simulink model "s5b"  (Simulink 2.00)
settings: Solver=ode15s  StartTime=0.0  StopTime=tstop  MaxStep=5e-3  RelTol=5e-6  AbsTol=1e-6
values from neighbouring files (symbols this model uses):
  Domega = 0    [P1HP.M]    (also in PSPH.M)
  H = J*wbm*wbm/(2*Sb)    (= 2.36870505626)    [P1HP.M]    (also in PSPH.M = 1.39074103839)
  Psidso = 0    [M1.M]    (also in M4.M; M4STP.M; M5.M)
  Psipdro = 0    [M1.M]    (also in M4.M; M4STP.M; M5.M; M6.M)
  Psipqro = 0    [M1.M]    (also in M4.M = Vm; M4STP.M = Vm; M5.M; M6.M)
  Psiqso = 0    [M1.M]    (also in M4.M = Vm; M4STP.M = Vm; M5.M; M6.M)
  rpr = 1.99    [P1HP.M]    (also in PSPH.M = 4.12)
  rs = 3.35    [P1HP.M]
  Tb = Sb/wbm    (= 3.9788735773)    [P1HP.M]    (also in PSPH.M = 0.989413229555)
  Tfactor = (3*P)/(4*wb)    (= 0.00795774715459)    [P1HP.M]    (also in PSPH.M = 0.00530516476973)
  Vm = Vrated*sqrt(2/3)    [M4.M]    (also in P1HP.M; PSPH.M = Vrated*sqrt(2))
  wb = 2*pi*frated    (= 376.991118431)    [P1HP.M]    (also in PSPH.M)
  wrbywbo = 0    [M1.M]    (also in M4.M = 1; M4STP.M = 1; M5.M; M6.M)
  xls = 6.94e-3*wb    (= 2.61631836191)    [P1HP.M]
  xM = 1/(1/xm + 1/xls + 1/xplr)    (= 1.2810101836)    [P1HP.M]
  xplr = xls    (= 2.61631836191)    [P1HP.M]    (also in PSPH.M = 2.12)
  Zb = Vrated*Vrated/Sb    (= 53.3333333333)    [P1HP.M]    (also in PSPH.M = 64.8793565684)
settings Model: MaxOrder=3  SaveTime=off  SaveOutput=off  ConsistencyChecking=off

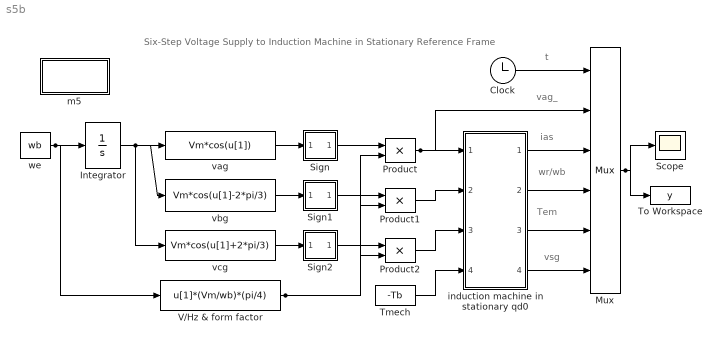
== system s5b ==
  note: Six-Step Voltage Supply to Induction Machine
      | in Stationary Reference Frame
  note: wr/wb
  note: Tem
  note: vsg
  note: ias
  note: vag_
  note: t
  Clock : Clock
      settings: DeleteFcn=simclock BlockIsBeingDestroyed  PostSaveFcn=simclock Save
  Integrator : Integrator  ExternalReset=none  InitialConditionSource=internal  InitialCondition=0  LimitOutput=off  UpperSaturationLimit=inf  LowerSaturationLimit=-inf  ShowSaturationPort=off  ShowStatePort=off  AbsoluteTolerance=auto
  m5 : Subsystem
      settings: OpenFcn=m5
      mask Type: Masked block of m5.m
      mask Help: Uses m5.5 to initialize and plot
      mask Display: disp('Initialize\nand plot')
  Mux : Mux  Inputs=6
  Product : Product  Inputs=2
  Product1 : Product  Inputs=2
  Product2 : Product  Inputs=2
  Scope : Scope
      settings: TickLabels=on  TimeRange=2  YMin=-20  YMax=20  SaveToWorkspace=off  SaveName=ScopeData  LimitMaxRows=off  Decimation=2
  Sign : Subsystem
      mask Type: Sign
      mask Description: y = sign(x)
      mask Help: Sign Function:\n\t\t\ty = 1 if x > 0\n\t\t\ty = 0 if x = 0\n\t\t\ty = -1 if x < 0
      mask Display: plot(-50,-50,50,50,[-50,50],[0,0],[0,0],[-50,50],[-40,0],[-30,-30],[0,40],[30,30])
  Sign1 : Subsystem
      mask Type: Sign
      mask Description: y = sign(x)
      mask Help: Sign Function:\n\t\t\ty = 1 if x > 0\n\t\t\ty = 0 if x = 0\n\t\t\ty = -1 if x < 0
      mask Display: plot(-50,-50,50,50,[-50,50],[0,0],[0,0],[-50,50],[-40,0],[-30,-30],[0,40],[30,30])
  Sign2 : Subsystem
      mask Type: Sign
      mask Description: y = sign(x)
      mask Help: Sign Function:\n\t\t\ty = 1 if x > 0\n\t\t\ty = 0 if x = 0\n\t\t\ty = -1 if x < 0
      mask Display: plot(-50,-50,50,50,[-50,50],[0,0],[0,0],[-50,50],[-40,0],[-30,-30],[0,40],[30,30])
  Tmech : Constant  Value=-Tb
  To Workspace : ToWorkspace  VariableName=y  SampleTime=0
      settings: Buffer=50000
  V/Hz & form factor : Fcn  Expr=u[1]*(Vm/wb)*(pi/4)
  induction machine in stationary qd0 : Subsystem
  vag : Fcn  Expr=Vm*cos(u[1])
  vbg : Fcn  Expr=Vm*cos(u[1]-2*pi/3)
  vcg : Fcn  Expr=Vm*cos(u[1]+2*pi/3)
  we : Constant  Value=wb
  wires:
  V/Hz & form factor/1 -> Product1/2, Product/2, Product2/2
  we/1 -> V/Hz & form factor/1, Integrator/1
  vcg/1 -> Sign2/1(in_1)
  vbg/1 -> Sign1/1(in_1)
  vag/1 -> Sign/1(in_1)
  Integrator/1 -> vbg/1, vag/1, vcg/1
  induction machine in stationary qd0/4(out_vsg) -> Mux/6
  induction machine in stationary qd0/3(out_Tem) -> Mux/5
  induction machine in stationary qd0/2(out_wr/wb) -> Mux/4
  induction machine in stationary qd0/1(out_ias) -> Mux/3
  Tmech/1 -> induction machine in stationary qd0/4(in_Tmech)
  Product/1 -> Mux/2, induction machine in stationary qd0/1(in_vag)
  Sign2/1(out_1) -> Product2/1
  Sign1/1(out_1) -> Product1/1
  Sign/1(out_1) -> Product/1
  Product2/1 -> induction machine in stationary qd0/3(in_vcg)
  Product1/1 -> induction machine in stationary qd0/2(in_vbg)
  Clock/1 -> Mux/1
  Mux/1 -> Scope/1, To Workspace/1

== system s5b/m5 ==
  note: Uses m5.m to initIalize simulation
      | and plot results

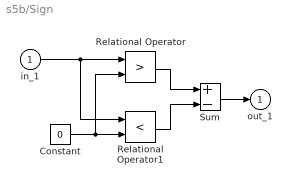
== system s5b/Sign ==
  in_1 : Inport  Port=1  PortWidth=-1  SampleTime=-1
  Constant : Constant  Value=0
  Relational Operator : RelationalOperator  Operator=>
  Relational Operator1 : RelationalOperator  Operator=<
  Sum : Sum  Inputs=+-
  out_1 : Outport  Port=1  InitialOutput=0
  wires:
  Sum/1 -> out_1/1
  Relational Operator/1 -> Sum/1
  Relational Operator1/1 -> Sum/2
  Constant/1 -> Relational Operator/2, Relational Operator1/2
  in_1/1 -> Relational Operator1/1, Relational Operator/1

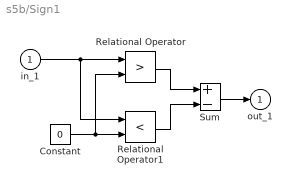
== system s5b/Sign1 ==
  in_1 : Inport  Port=1  PortWidth=-1  SampleTime=-1
  Constant : Constant  Value=0
  Relational Operator : RelationalOperator  Operator=>
  Relational Operator1 : RelationalOperator  Operator=<
  Sum : Sum  Inputs=+-
  out_1 : Outport  Port=1  InitialOutput=0
  wires:
  Sum/1 -> out_1/1
  Relational Operator/1 -> Sum/1
  Relational Operator1/1 -> Sum/2
  Constant/1 -> Relational Operator/2, Relational Operator1/2
  in_1/1 -> Relational Operator1/1, Relational Operator/1

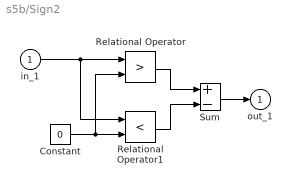
== system s5b/Sign2 ==
  in_1 : Inport  Port=1  PortWidth=-1  SampleTime=-1
  Constant : Constant  Value=0
  Relational Operator : RelationalOperator  Operator=>
  Relational Operator1 : RelationalOperator  Operator=<
  Sum : Sum  Inputs=+-
  out_1 : Outport  Port=1  InitialOutput=0
  wires:
  Sum/1 -> out_1/1
  Relational Operator/1 -> Sum/1
  Relational Operator1/1 -> Sum/2
  Constant/1 -> Relational Operator/2, Relational Operator1/2
  in_1/1 -> Relational Operator1/1, Relational Operator/1

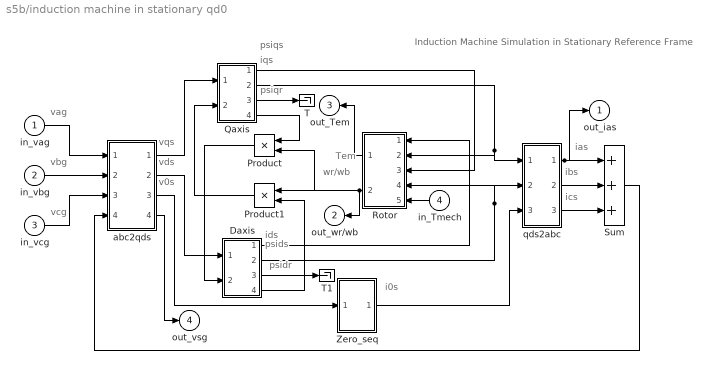
== system s5b/induction machine in stationary qd0 ==
  note: vbg
  note: ids
  note: v0s
  note: vds
  note: vqs
  note: ias
  note: psidr
  note: psids
  note: ics
  note: ibs
  note: psiqr
  note: iqs
  note: psiqs
  note: wr/wb
  note: Tem
  note: vcg
  note: vag
  note: i0s
  note: Induction Machine Simulation
      |   in Stationary Reference Frame
  in_vag : Inport  Port=1  PortWidth=-1  SampleTime=-1
  in_vbg : Inport  Port=2  PortWidth=-1  SampleTime=-1
  in_vcg : Inport  Port=3  PortWidth=-1  SampleTime=-1
  in_Tmech : Inport  Orientation=left  Port=4  PortWidth=-1  SampleTime=-1
  Daxis : Subsystem
  Product : Product  Orientation=left  Inputs=2
  Product1 : Product  Orientation=left  Inputs=2
  Qaxis : Subsystem
  Rotor : Subsystem  Orientation=left
  Sum : Sum  Inputs=+++
  T : Terminator
  T1 : Terminator
  Zero_seq : Subsystem
  abc2qds : Subsystem
  qds2abc : Subsystem
  out_ias : Outport  Port=1  InitialOutput=0
  out_wr/wb : Outport  Orientation=left  Port=2  InitialOutput=0
  out_Tem : Outport  Orientation=left  Port=3  InitialOutput=0
  out_vsg : Outport  Port=4  InitialOutput=0
  wires:
  Daxis/3(out_idr') -> T1/1
  Qaxis/3(out_iqr') -> T/1
  abc2qds/4(out_vsg) -> out_vsg/1
  in_Tmech/1 -> Rotor/5(in_Tmech)
  in_vcg/1 -> abc2qds/3(in_vcg)
  in_vbg/1 -> abc2qds/2(in_vbg)
  qds2abc/1(out_ias) -> out_ias/1, Sum/1
  Rotor/1(out_Tem) -> out_Tem/1
  in_vag/1 -> abc2qds/1(in_vag)
  Daxis/2(out_ids) -> Rotor/4(in_ids), qds2abc/2(in_ids)
  Product1/1 -> Qaxis/2(in_(wr/wb)*psidr')
  Qaxis/1(out_psiqs) -> Rotor/3(in_psiqs)
  abc2qds/2(out_vds) -> Daxis/1(in_vds)
  abc2qds/1(out_vqs) -> Qaxis/1(in_vqs)
  Qaxis/2(out_iqs) -> Rotor/2(in_iqs), qds2abc/1(in_iqs)
  Product/1 -> Daxis/2(in_(wr/wb)*psiqr')
  Daxis/1(out_psids) -> Rotor/1(in_psids)
  Rotor/2(out_wr/wb) -> out_wr/wb/1, Product/2, Product1/1
  Qaxis/4(out_psiqr') -> Product/1
  Daxis/4(out_psidr') -> Product1/2
  abc2qds/3(out_v0s) -> Zero_seq/1(in_v0s)
  qds2abc/2(out_ibs) -> Sum/2
  qds2abc/3(out_ics) -> Sum/3
  Zero_seq/1(out_i0s) -> qds2abc/3(in_i0s)
  Sum/1 -> abc2qds/4(ias+ibs+ics)

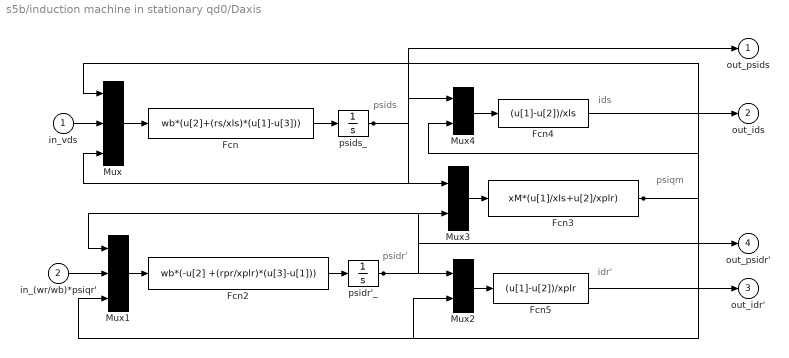
== system s5b/induction machine in stationary qd0/Daxis ==
  note: psidr'
  note: idr'
  note: psiqm
  note: psids
  note: ids
  in_vds : Inport  Port=1  PortWidth=-1  SampleTime=-1
  in_(wr/wb)*psiqr' : Inport  Port=2  PortWidth=-1  SampleTime=-1
  Fcn : Fcn  Expr=wb*(u[2]+(rs/xls)*(u[1]-u[3]))
  Fcn2 : Fcn  Expr=wb*(-u[2] +(rpr/xplr)*(u[3]-u[1]))
  Fcn3 : Fcn  Expr=xM*(u[1]/xls+u[2]/xplr)
  Fcn4 : Fcn  Expr=(u[1]-u[2])/xls
  Fcn5 : Fcn  Expr=(u[1]-u[2])/xplr
  Mux : Mux  Inputs=3
  Mux1 : Mux  Inputs=3
  Mux2 : Mux  Inputs=2
  Mux3 : Mux  Inputs=2
  Mux4 : Mux  Inputs=2
  psidr'_ : Integrator  ExternalReset=none  InitialConditionSource=internal  InitialCondition=Psipdro  LimitOutput=off  UpperSaturationLimit=inf  LowerSaturationLimit=-inf  ShowSaturationPort=off  ShowStatePort=off  AbsoluteTolerance=auto
  psids_ : Integrator  ExternalReset=none  InitialConditionSource=internal  InitialCondition=Psidso  LimitOutput=off  UpperSaturationLimit=inf  LowerSaturationLimit=-inf  ShowSaturationPort=off  ShowStatePort=off  AbsoluteTolerance=auto
  out_psids : Outport  Port=1  InitialOutput=0
  out_ids : Outport  Port=2  InitialOutput=0
  out_idr' : Outport  Port=3  InitialOutput=0
  out_psidr' : Outport  Port=4  InitialOutput=0
  wires:
  Fcn5/1 -> out_idr'/1
  in_(wr/wb)*psiqr'/1 -> Mux1/2
  in_vds/1 -> Mux/2
  Fcn4/1 -> out_ids/1
  Mux/1 -> Fcn/1
  Fcn/1 -> psids_/1
  Fcn2/1 -> psidr'_/1
  Mux3/1 -> Fcn3/1
  Mux4/1 -> Fcn4/1
  psids_/1 -> out_psids/1, Mux3/1, Mux4/1, Mux/3
  Fcn3/1 -> Mux4/2, Mux1/3, Mux/1, Mux2/2
  Mux1/1 -> Fcn2/1
  psidr'_/1 -> out_psidr'/1, Mux1/1, Mux3/2, Mux2/1
  Mux2/1 -> Fcn5/1

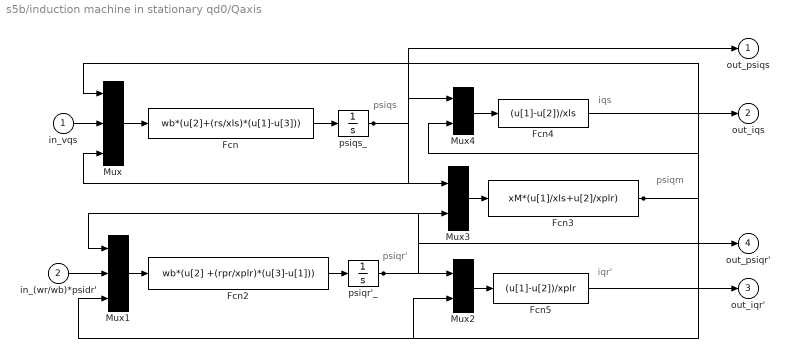
== system s5b/induction machine in stationary qd0/Qaxis ==
  note: psiqr'
  note: iqr'
  note: psiqm
  note: psiqs
  note: iqs
  in_vqs : Inport  Port=1  PortWidth=-1  SampleTime=-1
  in_(wr/wb)*psidr' : Inport  Port=2  PortWidth=-1  SampleTime=-1
  Fcn : Fcn  Expr=wb*(u[2]+(rs/xls)*(u[1]-u[3]))
  Fcn2 : Fcn  Expr=wb*(u[2] +(rpr/xplr)*(u[3]-u[1]))
  Fcn3 : Fcn  Expr=xM*(u[1]/xls+u[2]/xplr)
  Fcn4 : Fcn  Expr=(u[1]-u[2])/xls
  Fcn5 : Fcn  Expr=(u[1]-u[2])/xplr
  Mux : Mux  Inputs=3
  Mux1 : Mux  Inputs=3
  Mux2 : Mux  Inputs=2
  Mux3 : Mux  Inputs=2
  Mux4 : Mux  Inputs=2
  psiqr'_ : Integrator  ExternalReset=none  InitialConditionSource=internal  InitialCondition=Psipqro  LimitOutput=off  UpperSaturationLimit=inf  LowerSaturationLimit=-inf  ShowSaturationPort=off  ShowStatePort=off  AbsoluteTolerance=auto
  psiqs_ : Integrator  ExternalReset=none  InitialConditionSource=internal  InitialCondition=Psiqso  LimitOutput=off  UpperSaturationLimit=inf  LowerSaturationLimit=-inf  ShowSaturationPort=off  ShowStatePort=off  AbsoluteTolerance=auto
  out_psiqs : Outport  Port=1  InitialOutput=0
  out_iqs : Outport  Port=2  InitialOutput=0
  out_iqr' : Outport  Port=3  InitialOutput=0
  out_psiqr' : Outport  Port=4  InitialOutput=0
  wires:
  Fcn5/1 -> out_iqr'/1
  in_(wr/wb)*psidr'/1 -> Mux1/2
  in_vqs/1 -> Mux/2
  Fcn4/1 -> out_iqs/1
  Mux/1 -> Fcn/1
  Fcn/1 -> psiqs_/1
  Fcn2/1 -> psiqr'_/1
  Mux3/1 -> Fcn3/1
  Mux4/1 -> Fcn4/1
  psiqs_/1 -> out_psiqs/1, Mux3/1, Mux4/1, Mux/3
  Fcn3/1 -> Mux4/2, Mux1/3, Mux/1, Mux2/2
  Mux1/1 -> Fcn2/1
  psiqr'_/1 -> out_psiqr'/1, Mux1/1, Mux3/2, Mux2/1
  Mux2/1 -> Fcn5/1

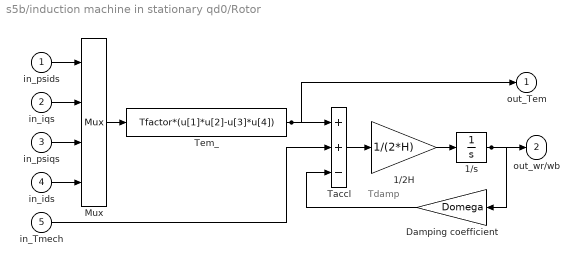
== system s5b/induction machine in stationary qd0/Rotor ==
  note: Tdamp
  in_psids : Inport  Port=1  PortWidth=-1  SampleTime=-1
  in_iqs : Inport  Port=2  PortWidth=-1  SampleTime=-1
  in_psiqs : Inport  Port=3  PortWidth=-1  SampleTime=-1
  in_ids : Inport  Port=4  PortWidth=-1  SampleTime=-1
  in_Tmech : Inport  Port=5  PortWidth=-1  SampleTime=-1
  1/2H : Gain  Gain=1/(2*H)
  1/s : Integrator  ExternalReset=none  InitialConditionSource=internal  InitialCondition=wrbywbo  LimitOutput=off  UpperSaturationLimit=inf  LowerSaturationLimit=-inf  ShowSaturationPort=off  ShowStatePort=off  AbsoluteTolerance=auto
  Damping coefficient : Gain  Orientation=left  Gain=Domega
  Mux : Mux  Inputs=4
  Taccl : Sum  Inputs=++-
  Tem_ : Fcn  Expr=Tfactor*(u[1]*u[2]-u[3]*u[4])
  out_Tem : Outport  Port=1  InitialOutput=0
  out_wr/wb : Outport  Port=2  InitialOutput=0
  wires:
  in_ids/1 -> Mux/4
  in_psiqs/1 -> Mux/3
  in_iqs/1 -> Mux/2
  in_psids/1 -> Mux/1
  Mux/1 -> Tem_/1
  Damping coefficient/1 -> Taccl/3
  1/s/1 -> Damping coefficient/1, out_wr/wb/1
  Tem_/1 -> out_Tem/1, Taccl/1
  1/2H/1 -> 1/s/1
  Taccl/1 -> 1/2H/1
  in_Tmech/1 -> Taccl/2

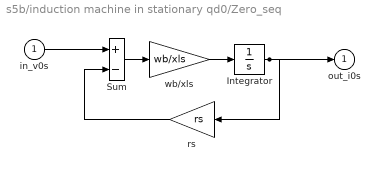
== system s5b/induction machine in stationary qd0/Zero_seq ==
  in_v0s : Inport  Port=1  PortWidth=-1  SampleTime=-1
  Integrator : Integrator  ExternalReset=none  InitialConditionSource=internal  InitialCondition=0  LimitOutput=off  UpperSaturationLimit=inf  LowerSaturationLimit=-inf  ShowSaturationPort=off  ShowStatePort=off  AbsoluteTolerance=auto
  Sum : Sum  Inputs=+-
  rs : Gain  Orientation=left  Gain=rs
  wb/xls : Gain  Gain=wb/xls
  out_i0s : Outport  Port=1  InitialOutput=0
  wires:
  Integrator/1 -> out_i0s/1, rs/1
  in_v0s/1 -> Sum/1
  wb/xls/1 -> Integrator/1
  Sum/1 -> wb/xls/1
  rs/1 -> Sum/2

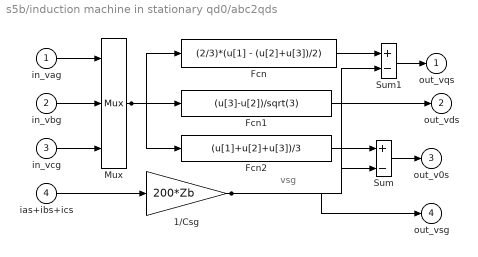
== system s5b/induction machine in stationary qd0/abc2qds ==
  note: vsg
  in_vag : Inport  Port=1  PortWidth=-1  SampleTime=-1
  in_vbg : Inport  Port=2  PortWidth=-1  SampleTime=-1
  in_vcg : Inport  Port=3  PortWidth=-1  SampleTime=-1
  ias+ibs+ics : Inport  Port=4  PortWidth=-1  SampleTime=-1
  1/Csg : Gain  Gain=200*Zb
  Fcn : Fcn  Expr=(2/3)*(u[1] - (u[2]+u[3])/2)
  Fcn1 : Fcn  Expr=(u[3]-u[2])/sqrt(3)
  Fcn2 : Fcn  Expr=(u[1]+u[2]+u[3])/3
  Mux : Mux  Inputs=3
  Sum : Sum  Inputs=+-
  Sum1 : Sum  Inputs=+-
  out_vqs : Outport  Port=1  InitialOutput=0
  out_vds : Outport  Port=2  InitialOutput=0
  out_v0s : Outport  Port=3  InitialOutput=0
  out_vsg : Outport  Port=4  InitialOutput=0
  wires:
  1/Csg/1 -> Sum1/2, out_vsg/1, Sum/2
  Sum1/1 -> out_vqs/1
  Fcn/1 -> Sum1/1
  ias+ibs+ics/1 -> 1/Csg/1
  Fcn2/1 -> Sum/1
  Sum/1 -> out_v0s/1
  Fcn1/1 -> out_vds/1
  Mux/1 -> Fcn2/1, Fcn/1, Fcn1/1
  in_vcg/1 -> Mux/3
  in_vbg/1 -> Mux/2
  in_vag/1 -> Mux/1

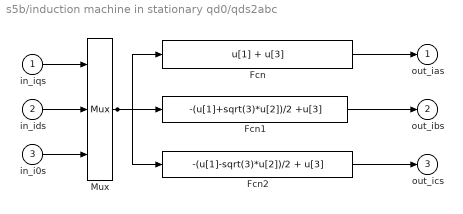
== system s5b/induction machine in stationary qd0/qds2abc ==
  in_iqs : Inport  Port=1  PortWidth=-1  SampleTime=-1
  in_ids : Inport  Port=2  PortWidth=-1  SampleTime=-1
  in_i0s : Inport  Port=3  PortWidth=-1  SampleTime=-1
  Fcn : Fcn  Expr=u[1] + u[3]
  Fcn1 : Fcn  Expr=-(u[1]+sqrt(3)*u[2])/2 +u[3]
  Fcn2 : Fcn  Expr=-(u[1]-sqrt(3)*u[2])/2 + u[3]
  Mux : Mux  Inputs=3
  out_ias : Outport  Port=1  InitialOutput=0
  out_ibs : Outport  Port=2  InitialOutput=0
  out_ics : Outport  Port=3  InitialOutput=0
  wires:
  Fcn2/1 -> out_ics/1
  Mux/1 -> Fcn2/1, Fcn/1, Fcn1/1
  Fcn/1 -> out_ias/1
  Fcn1/1 -> out_ibs/1
  in_i0s/1 -> Mux/3
  in_iqs/1 -> Mux/1
  in_ids/1 -> Mux/2
